simulink model "MOBATSim"  (R2020b)
settings: Solver=FixedStepAuto  StartTime=0.0  StopTime=Sim_t  FixedStep=0.005  MinStep=0.01  RelTol=1e-2
undefined symbols (not defined in the file): FIBlock, FIBlockLib, meters, Sim_Ts, Vehicle_id, Vehicles
libraries: simulink x31, robotalgslib x11, drivingvehiclecontroller x11, mpcadaslib x1, pid_lib x1
(part 6 of 6)

== system MOBATSim/Vehicle Model 9/Longitudinal and Lateral Controllers/Lateral Motion Control/Pure Pursuit/Wheel Steering Angle Formulation ==
  note: $\delta(t)=tan^{-1} \left( \frac{2\ L\ sin(\alpha)}{l_{d}} \right)$
  alpha : Inport
  Atan : Trigonometry  Operator=atan
  Divide : Product  Inputs=*/
  Gain : Gain  Gain=2
  One over Look Ahead Distance : Constant  Value=6
  Product : Product
  Sine Wave : Sin  TimeSource=Use external signal  SampleTime=0
  Wheel Base : Constant  Value=3
  referenceYawAngle : Outport
  wires:
  Wheel Base/1 -> Gain/1
  Gain/1 -> Product/1
  alpha/1 -> Sine Wave/1
  Sine Wave/1 -> Product/2
  Product/1 -> Divide/1
  One over Look Ahead Distance/1 -> Divide/2
  Divide/1 -> Atan/1
  Atan/1 -> referenceYawAngle/1

== stateflow chart MOBATSim/Vehicle Model 6/Longitudinal and Lateral Controllers/Longitudinal Speed Control/Reference Acceleration Generation/Gear Logic ==
  settings: sampleTime=0.1
  state Gear1
    entry:
    maxAcc=6;
  state Gear2
    entry:
    maxAcc=5;
  state Gear3
    entry:
    maxAcc=3.8;
  state Gear4
    entry:
    maxAcc=3;
  state Gear5
    entry:
    maxAcc=2.2;
  state Gear6
    entry:
    maxAcc=1.4;
  (default) -> Gear1
  Gear3 -> Gear4 [order 2] : [speed>9]
  Gear4 -> Gear5 [order 1] : [speed>12]
  Gear2 -> Gear3 [order 1] : [speed>6]
  Gear5 -> Gear6 [order 2] : [speed>14]
  Gear1 -> Gear2 : [speed>3]
  Gear6 -> Gear5 : [speed<14]
  Gear4 -> Gear3 [order 2] : [speed<9]
  Gear5 -> Gear4 [order 1] : [speed<12]
  Gear2 -> Gear1 [order 2] : [speed<3]
  Gear3 -> Gear2 [order 1] : [speed<6]
  data: speed input; maxAcc output

== stateflow chart MOBATSim/Vehicle Model 7/Longitudinal and Lateral Controllers/Longitudinal Speed Control/Reference Acceleration Generation/Gear Logic ==
  settings: sampleTime=0.1
  state Gear1
    entry:
    maxAcc=6;
  state Gear2
    entry:
    maxAcc=5;
  state Gear3
    entry:
    maxAcc=3.8;
  state Gear4
    entry:
    maxAcc=3;
  state Gear5
    entry:
    maxAcc=2.2;
  state Gear6
    entry:
    maxAcc=1.4;
  (default) -> Gear1
  Gear3 -> Gear4 [order 2] : [speed>9]
  Gear4 -> Gear5 [order 1] : [speed>12]
  Gear2 -> Gear3 [order 1] : [speed>6]
  Gear5 -> Gear6 [order 2] : [speed>14]
  Gear1 -> Gear2 : [speed>3]
  Gear6 -> Gear5 : [speed<14]
  Gear4 -> Gear3 [order 2] : [speed<9]
  Gear5 -> Gear4 [order 1] : [speed<12]
  Gear2 -> Gear1 [order 2] : [speed<3]
  Gear3 -> Gear2 [order 1] : [speed<6]
  data: speed input; maxAcc output

== stateflow chart MOBATSim/Vehicle Model 8/Longitudinal and Lateral Controllers/Longitudinal Speed Control/Reference Acceleration Generation/Gear Logic ==
  settings: sampleTime=0.1
  state Gear1
    entry:
    maxAcc=6;
  state Gear2
    entry:
    maxAcc=5;
  state Gear3
    entry:
    maxAcc=3.8;
  state Gear4
    entry:
    maxAcc=3;
  state Gear5
    entry:
    maxAcc=2.2;
  state Gear6
    entry:
    maxAcc=1.4;
  (default) -> Gear1
  Gear3 -> Gear4 [order 2] : [speed>9]
  Gear4 -> Gear5 [order 1] : [speed>12]
  Gear2 -> Gear3 [order 1] : [speed>6]
  Gear5 -> Gear6 [order 2] : [speed>14]
  Gear1 -> Gear2 : [speed>3]
  Gear6 -> Gear5 : [speed<14]
  Gear4 -> Gear3 [order 2] : [speed<9]
  Gear5 -> Gear4 [order 1] : [speed<12]
  Gear2 -> Gear1 [order 2] : [speed<3]
  Gear3 -> Gear2 [order 1] : [speed<6]
  data: speed input; maxAcc output

== stateflow chart MOBATSim/Vehicle Model 9/Longitudinal and Lateral Controllers/Longitudinal Speed Control/Reference Acceleration Generation/Gear Logic ==
  settings: sampleTime=0.1
  state Gear1
    entry:
    maxAcc=6;
  state Gear2
    entry:
    maxAcc=5;
  state Gear3
    entry:
    maxAcc=3.8;
  state Gear4
    entry:
    maxAcc=3;
  state Gear5
    entry:
    maxAcc=2.2;
  state Gear6
    entry:
    maxAcc=1.4;
  (default) -> Gear1
  Gear3 -> Gear4 [order 2] : [speed>9]
  Gear4 -> Gear5 [order 1] : [speed>12]
  Gear2 -> Gear3 [order 1] : [speed>6]
  Gear5 -> Gear6 [order 2] : [speed>14]
  Gear1 -> Gear2 : [speed>3]
  Gear6 -> Gear5 : [speed<14]
  Gear4 -> Gear3 [order 2] : [speed<9]
  Gear5 -> Gear4 [order 1] : [speed<12]
  Gear2 -> Gear1 [order 2] : [speed<3]
  Gear3 -> Gear2 [order 1] : [speed<6]
  data: speed input; maxAcc output

== stateflow chart MOBATSim/Vehicle Model 10/Longitudinal and Lateral Controllers/Longitudinal Speed Control/Reference Acceleration Generation/Gear Logic ==
  settings: sampleTime=0.1
  state Gear1
    entry:
    maxAcc=6;
  state Gear2
    entry:
    maxAcc=5;
  state Gear3
    entry:
    maxAcc=3.8;
  state Gear4
    entry:
    maxAcc=3;
  state Gear5
    entry:
    maxAcc=2.2;
  state Gear6
    entry:
    maxAcc=1.4;
  (default) -> Gear1
  Gear3 -> Gear4 [order 2] : [speed>9]
  Gear4 -> Gear5 [order 1] : [speed>12]
  Gear2 -> Gear3 [order 1] : [speed>6]
  Gear5 -> Gear6 [order 2] : [speed>14]
  Gear1 -> Gear2 : [speed>3]
  Gear6 -> Gear5 : [speed<14]
  Gear4 -> Gear3 [order 2] : [speed<9]
  Gear5 -> Gear4 [order 1] : [speed<12]
  Gear2 -> Gear1 [order 2] : [speed<3]
  Gear3 -> Gear2 [order 1] : [speed<6]
  data: speed input; maxAcc output

== matlab function MOBATSim/Vehicle Model 2/FIBlock2/FaultInjectionBlock ==
  data: time input; error_data output; data input; input_flag input; FIBlockName parameter; error_flag output
function [error_data, error_flag] = fcn(time, data, input_flag, FIBlockName)
coder.extrinsic('wrapper');
d = data;
t = time;
n = num2str(FIBlockName);
f = input_flag;
error_data = coder.nullcopy(zeros(size(d)));
error_flag = 0;
[error_data, error_flag] = wrapper(d, t, n, f);
end

== matlab function MOBATSim/Vehicle Model 2/FIBlock1/FaultInjectionBlock ==
  data: time input; error_data output; data input; input_flag input; FIBlockName parameter; error_flag output
function [error_data, error_flag] = fcn(time, data, input_flag, FIBlockName)
coder.extrinsic('wrapper');
d = data;
t = time;
n = num2str(FIBlockName);
f = input_flag;
error_data = coder.nullcopy(zeros(size(d)));
error_flag = 0;
[error_data, error_flag] = wrapper(d, t, n, f);
end

== matlab function MOBATSim/Vehicle Model 6/FIBlock/FaultInjectionBlock ==
  data: time input; error_data output; data input; input_flag input; FIBlockName parameter; error_flag output
function [error_data, error_flag] = fcn(time, data, input_flag, FIBlockName)
coder.extrinsic('wrapper');
d = data;
t = time;
n = num2str(FIBlockName);
f = input_flag;
error_data = coder.nullcopy(zeros(size(d)));
error_flag = 0;
[error_data, error_flag] = wrapper(d, t, n, f);
end

== matlab function MOBATSim/Vehicle Model 6/FIBlock1/FaultInjectionBlock ==
  data: time input; error_data output; data input; input_flag input; FIBlockName parameter; error_flag output
function [error_data, error_flag] = fcn(time, data, input_flag, FIBlockName)
coder.extrinsic('wrapper');
d = data;
t = time;
n = num2str(FIBlockName);
f = input_flag;
error_data = coder.nullcopy(zeros(size(d)));
error_flag = 0;
[error_data, error_flag] = wrapper(d, t, n, f);
end

== stateflow chart MOBATSim/Vehicle Model 2/Longitudinal and Lateral Controllers/Longitudinal Speed Control/Reference Acceleration Generation/Gear Logic ==
  settings: sampleTime=0.1
  state Gear1
    entry:
    maxAcc=6;
  state Gear2
    entry:
    maxAcc=5;
  state Gear3
    entry:
    maxAcc=3.8;
  state Gear4
    entry:
    maxAcc=3;
  state Gear5
    entry:
    maxAcc=2.2;
  state Gear6
    entry:
    maxAcc=1.4;
  (default) -> Gear1
  Gear3 -> Gear4 [order 2] : [speed>9]
  Gear4 -> Gear5 [order 1] : [speed>12]
  Gear2 -> Gear3 [order 1] : [speed>6]
  Gear5 -> Gear6 [order 2] : [speed>14]
  Gear1 -> Gear2 : [speed>3]
  Gear6 -> Gear5 : [speed<14]
  Gear4 -> Gear3 [order 2] : [speed<9]
  Gear5 -> Gear4 [order 1] : [speed<12]
  Gear2 -> Gear1 [order 2] : [speed<3]
  Gear3 -> Gear2 [order 1] : [speed<6]
  data: speed input; maxAcc output

== stateflow chart MOBATSim/Vehicle Model 1/Longitudinal and Lateral Controllers/Longitudinal Speed Control/Reference Acceleration Generation/Gear Logic ==
  settings: sampleTime=0.1
  state Gear1
    entry:
    maxAcc=6;
  state Gear2
    entry:
    maxAcc=5;
  state Gear3
    entry:
    maxAcc=3.8;
  state Gear4
    entry:
    maxAcc=3;
  state Gear5
    entry:
    maxAcc=2.2;
  state Gear6
    entry:
    maxAcc=1.4;
  (default) -> Gear1
  Gear3 -> Gear4 [order 2] : [speed>9]
  Gear4 -> Gear5 [order 1] : [speed>12]
  Gear2 -> Gear3 [order 1] : [speed>6]
  Gear5 -> Gear6 [order 2] : [speed>14]
  Gear1 -> Gear2 : [speed>3]
  Gear6 -> Gear5 : [speed<14]
  Gear4 -> Gear3 [order 2] : [speed<9]
  Gear5 -> Gear4 [order 1] : [speed<12]
  Gear2 -> Gear1 [order 2] : [speed<3]
  Gear3 -> Gear2 [order 1] : [speed<6]
  data: speed input; maxAcc output

== stateflow chart MOBATSim/Vehicle Model 3/Longitudinal and Lateral Controllers/Longitudinal Speed Control/Reference Acceleration Generation/Gear Logic ==
  settings: sampleTime=0.1
  state Gear1
    entry:
    maxAcc=6;
  state Gear2
    entry:
    maxAcc=5;
  state Gear3
    entry:
    maxAcc=3.8;
  state Gear4
    entry:
    maxAcc=3;
  state Gear5
    entry:
    maxAcc=2.2;
  state Gear6
    entry:
    maxAcc=1.4;
  (default) -> Gear1
  Gear3 -> Gear4 [order 2] : [speed>9]
  Gear4 -> Gear5 [order 1] : [speed>12]
  Gear2 -> Gear3 [order 1] : [speed>6]
  Gear5 -> Gear6 [order 2] : [speed>14]
  Gear1 -> Gear2 : [speed>3]
  Gear6 -> Gear5 : [speed<14]
  Gear4 -> Gear3 [order 2] : [speed<9]
  Gear5 -> Gear4 [order 1] : [speed<12]
  Gear2 -> Gear1 [order 2] : [speed<3]
  Gear3 -> Gear2 [order 1] : [speed<6]
  data: speed input; maxAcc output

== stateflow chart MOBATSim/Vehicle Model 4/Longitudinal and Lateral Controllers/Longitudinal Speed Control/Reference Acceleration Generation/Gear Logic ==
  settings: sampleTime=0.1
  state Gear1
    entry:
    maxAcc=6;
  state Gear2
    entry:
    maxAcc=5;
  state Gear3
    entry:
    maxAcc=3.8;
  state Gear4
    entry:
    maxAcc=3;
  state Gear5
    entry:
    maxAcc=2.2;
  state Gear6
    entry:
    maxAcc=1.4;
  (default) -> Gear1
  Gear3 -> Gear4 [order 2] : [speed>9]
  Gear4 -> Gear5 [order 1] : [speed>12]
  Gear2 -> Gear3 [order 1] : [speed>6]
  Gear5 -> Gear6 [order 2] : [speed>14]
  Gear1 -> Gear2 : [speed>3]
  Gear6 -> Gear5 : [speed<14]
  Gear4 -> Gear3 [order 2] : [speed<9]
  Gear5 -> Gear4 [order 1] : [speed<12]
  Gear2 -> Gear1 [order 2] : [speed<3]
  Gear3 -> Gear2 [order 1] : [speed<6]
  data: speed input; maxAcc output

== stateflow chart MOBATSim/Vehicle Model 5/Longitudinal and Lateral Controllers/Longitudinal Speed Control/Reference Acceleration Generation/Gear Logic ==
  settings: sampleTime=0.1
  state Gear1
    entry:
    maxAcc=6;
  state Gear2
    entry:
    maxAcc=5;
  state Gear3
    entry:
    maxAcc=3.8;
  state Gear4
    entry:
    maxAcc=3;
  state Gear5
    entry:
    maxAcc=2.2;
  state Gear6
    entry:
    maxAcc=1.4;
  (default) -> Gear1
  Gear3 -> Gear4 [order 2] : [speed>9]
  Gear4 -> Gear5 [order 1] : [speed>12]
  Gear2 -> Gear3 [order 1] : [speed>6]
  Gear5 -> Gear6 [order 2] : [speed>14]
  Gear1 -> Gear2 : [speed>3]
  Gear6 -> Gear5 : [speed<14]
  Gear4 -> Gear3 [order 2] : [speed<9]
  Gear5 -> Gear4 [order 1] : [speed<12]
  Gear2 -> Gear1 [order 2] : [speed<3]
  Gear3 -> Gear2 [order 1] : [speed<6]
  data: speed input; maxAcc output
